simulink model "helicoptertemplate_lqi_test_2"  (R2021b)
settings: Solver=ode45  StartTime=0.0  StopTime=Tsim  RelTol=1e-3
InitFcn:
  | hwinit
values from neighbouring files (symbols this model uses):
  adingain = [pitchgain 1 1 1]    [hwinit.m]
  adinoffs = [pitchoffs 0 0 0]    [hwinit.m]
  h = 0.01    [LQR_LQI_init.m]
  sysd = c2d(sys, h)    [LQR_LQI_init.m]
undefined symbols (not defined in the file or in its folder): DiscIntNeverNeededParam, Discrete, HeliMexHandle, Kd_i, Time
libraries: ctrlSharedLib x1, eeStairGenerator x1
settings Model: Creator=fkzhang  LastModifiedBy=rjvanderhorst
settings SolverCC: AlgebraicLoopSolver=TrustRegion
settings DataIOCC: LimitDataPoints=on  SaveFormat=Array  ReturnWorkspaceOutputs=off
settings OptimizationCC: BlockReduction=off  BooleanDataType=off  LifeSpan=inf
settings DebuggingCC: SaveWithParameterizedLinksMsg=none  UnderspecifiedInitializationDetection=Classic  MergeDetectMultiDrivingBlocksExec=none  SignalResolutionControl=TryResolveAllWithWarning  AllowSymbolicDim=off  SFUnexpectedBacktrackingDiag=warning  SFNoUnconditionalDefaultTransitionDiag=warning  SFExecutionAtInitializationDiag=none  SFMachineParentedDataDiag=warning  ArithmeticOperatorsInVariantConditions=warning
settings HardwareCC: ProdBitPerPointer=32  ProdBitPerSizeT=32  ProdBitPerPtrDiffT=32  ProdLargestAtomicFloat=None  ProdIntDivRoundTo=Undefined  ProdEndianess=Unspecified  ProdWordSize=32  ProdHWDeviceType=32-bit Generic  TargetUnknown=on
settings ModelReferenceCC: PropagateSignalLabelsOutOfModel=off
settings SFSimCC: SimUseLocalCustomCode=off  CustomCodeUndefinedFunction=UseInterfaceOnly
settings RTWCC: RTWUseLocalCustomCode=off
settings CodeAppCC: StateflowObjectComments=on
settings GRTTargetCC: TargetLangStandard=C89/C90 (ANSI)
settings ConfigComp: CovMetricSettings=dw  CovSaveCumulativeToWorkspaceVar=on  CovSaveSingleToWorkspaceVar=on  CovExternalEMLEnable=off  CovSFcnEnable=off

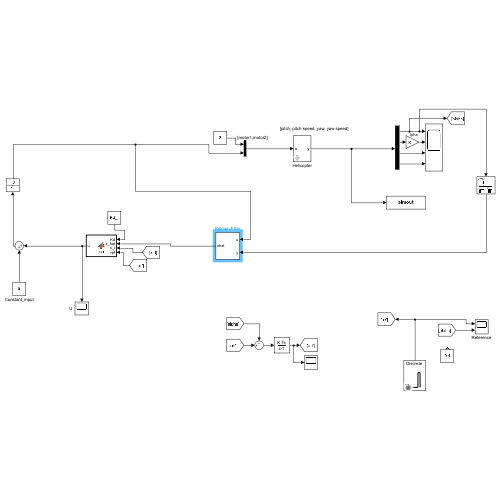
[thumbnail: Simulink's stored preview of the top-level diagram]
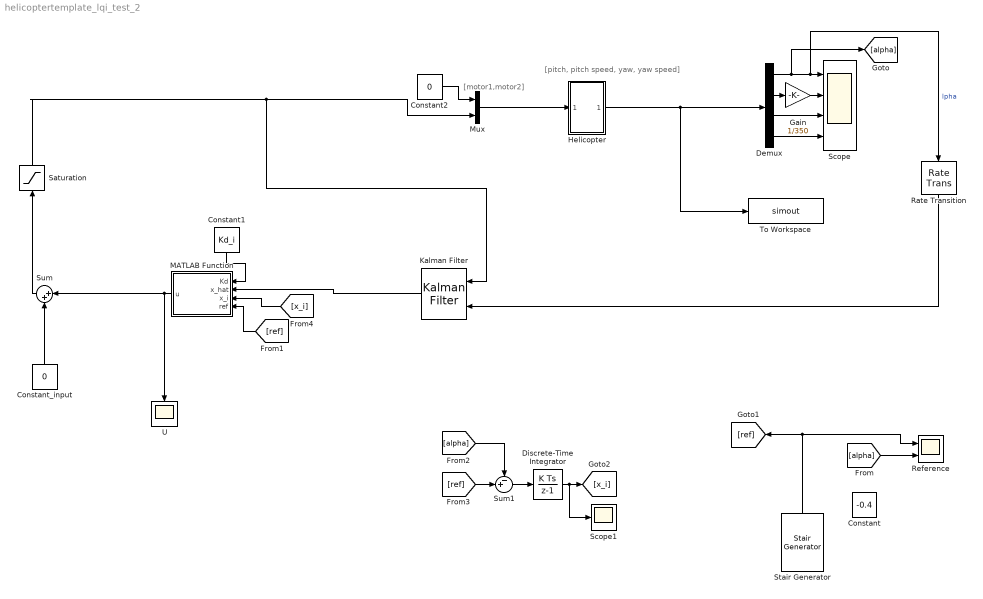
== system helicoptertemplate_lqi_test_2 ==
  note: [pitch, pitch speed, yaw, yaw speed]
  note: [motor1,motor2]
  Constant : Constant  Value=-0.4
  Constant1 : Constant  Value=Kd_i  LockScale=on
  Constant2 : Constant  Value=0
  Constant_input : Constant  Value=0
  Demux : Demux
  Discrete-Time Integrator : DiscreteIntegrator  SampleTime=-1  ICPrevOutput=DiscIntNeverNeededParam  ICPrevScaledInput=DiscIntNeverNeededParam
  Gain : Gain  Gain=1/350
  Helicopter : Subsystem  mask{Ts=h}
      mask prompts: Ts "sampletime"
      mask init:
      | sf_heli_init
      mask Display:
      | port_label('input',1,'u');
      | port_label('output',1,'y');
  Kalman Filter : ctrlSharedLib/Kalman Filter  TimeDomain=Discrete-Time  UseCurrentEstimator=on  ModelSource=Individual A, B, C, D matrices  ModelSourceVariable=ss(0.95,1,1,0,1)  A=sysd.A  B=sysd.B  C=sysd.C  D=sysd.D  NumberOfStates=1  NumberOfInputs=1  NumberOfOutputs=1  InitialEstimateSource=Dialog  X0=[0; 0]  P0=10  UseK=off  UseGH=off  NumberOfProcessNoiseInputs=1  G=1  TimeInvariantG=on  H=0  TimeInvariantH=on  Q=0.05  TimeInvariantQ=on  R=1  TimeInvariantR=on  N=0  TimeInvariantN=on  AddInputPort=on  AddEnablePort=off  OutputEstimatedY=off  OutputP=off  Ts=h
  MATLAB Function : MATLAB Function  TreatAsAtomicUnit=on
  Mux : Mux  Inputs=2
  Rate Transition : RateTransition  OutPortSampleTime=h
  Reference : Scope  NumInputPorts=2
  Saturation : Saturate  UpperLimit=1  LowerLimit=-1
  Scope : Scope  NumInputPorts=4
  Scope1 : Scope
  Stair Generator : eeStairGenerator/Stair Generator  LabelModeActiveChoice=Discrete  TimeInput=[0 20 40 50]  AmplitudeInput=[-0.1 -0.1 -0.05 -0.1]  SampleTime=h  RepeatPattern=off  OutDataTypeStr=double
      settings: SourceProductBaseCode=PS
  Sum : Sum  Inputs=|++
  Sum1 : Sum  Inputs=-+|
  To Workspace : ToWorkspace  VariableName=simout  SaveFormat=Structure With Time  SampleTime=-1
  U : Scope
  wires:
  Helicopter/1(Out1) -> To Workspace/1, Demux/1
  Mux/1 -> Helicopter/1(In1)
  Demux/3 -> Scope/3
  Demux/4 -> Scope/4
  Demux/2 -> Gain/1
  Gain/1 -> Scope/2
  Demux/1 -> [alpha], Rate Transition/1, Scope/1  "lpha"
  Constant1/1 -> MATLAB Function/1(Kd)
  Constant_input/1 -> Sum/2
  Sum/1 -> Saturation/1
  MATLAB Function/1(u) -> U/1, Sum/1
  Kalman Filter/1 -> MATLAB Function/2(x_hat)
  Saturation/1 -> Kalman Filter/1, Mux/2
  Rate Transition/1 -> Kalman Filter/2
  [alpha] -> Reference/2
  Stair Generator/1 -> [ref], Reference/1
  [ref] -> MATLAB Function/4(ref)
  [alpha] -> Sum1/1
  [ref] -> Sum1/2
  Sum1/1 -> Discrete-Time Integrator/1
  Discrete-Time Integrator/1 -> Scope1/1, [x_i]
  [x_i] -> MATLAB Function/3(x_i)
  Constant2/1 -> Mux/1

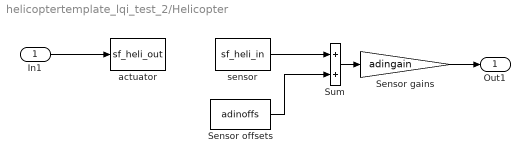
== system helicoptertemplate_lqi_test_2/Helicopter ==
  In1 : Inport
  Sensor gains : Gain  Gain=adingain
  Sensor offsets : Constant  Value=adinoffs
  Sum : Sum
  actuator : M-S-Function  FunctionName=sf_heli_out  Parameters=HeliMexHandle,Ts
  sensor : M-S-Function  FunctionName=sf_heli_in  Parameters=HeliMexHandle
  Out1 : Outport
  wires:
  sensor/1 -> Sum/1
  In1/1 -> actuator/1
  Sensor offsets/1 -> Sum/2
  Sum/1 -> Sensor gains/1
  Sensor gains/1 -> Out1/1

== matlab function helicoptertemplate_lqi_test_2/MATLAB Function ==
  data: Kd input; x_hat input; x_i input; u output; ref input
function u = fcn(Kd, x_hat, x_i, ref)
    x_ref = [ref; 0];
    error = x_hat-x_ref;
    state_vector = [error; x_i];
    u = (-Kd'*state_vector);
end
